simulink library "time_conversions_lib"  (R2016b)
settings: Solver=ode45  StartTime=0.0  StopTime=10.0  RelTol=1e-3  EnableMultiTasking=on
settings Model: Creator=Taylor  LastModifiedBy=Taylor
settings DataIOCC: LimitDataPoints=on
settings OptimizationCC: LifeSpan=inf
settings DebuggingCC: AllowSymbolicDim=off  SFUnexpectedBacktrackingDiag=warning  SFNoUnconditionalDefaultTransitionDiag=warning  SFExecutionAtInitializationDiag=none
settings GRTTargetCC: TargetLangStandard=C89/C90 (ANSI)  GeneratePreprocessorConditionals=Disable all
settings ConfigComp: CovMetricSettings=dw  CovHtmlReporting=on  CovSaveCumulativeToWorkspaceVar=on  CovSaveSingleToWorkspaceVar=on  CovExternalEMLEnable=off

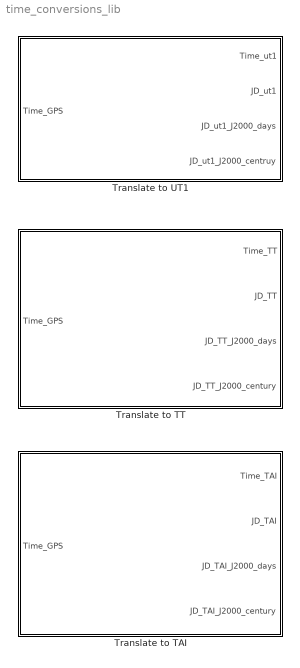
== system time_conversions_lib ==
  Translate to TAI : Subsystem
  Translate to TT : Subsystem
  Translate to UT1 : Subsystem

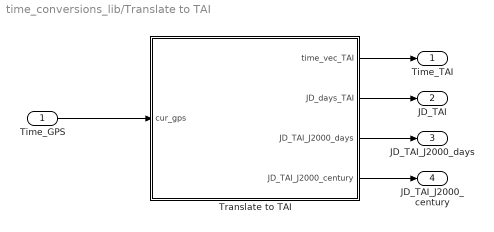
== system time_conversions_lib/Translate to TAI ==
  Time_GPS : Inport
  Translate to TAI : MATLAB Function  TreatAsAtomicUnit=on
  Time_TAI : Outport
  JD_TAI : Outport  Port=2
  JD_TAI_J2000_days : Outport  Port=3
  JD_TAI_J2000_century : Outport  Port=4
  wires:
  Translate to TAI/3(JD_TAI_J2000_days) -> JD_TAI_J2000_days/1
  Time_GPS/1 -> Translate to TAI/1(cur_gps)
  Translate to TAI/1(time_vec_TAI) -> Time_TAI/1
  Translate to TAI/2(JD_days_TAI) -> JD_TAI/1
  Translate to TAI/4(JD_TAI_J2000_century) -> JD_TAI_J2000_century/1

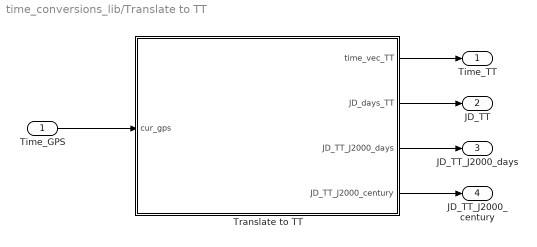
== system time_conversions_lib/Translate to TT ==
  Time_GPS : Inport
  Translate to TT : MATLAB Function  TreatAsAtomicUnit=on
  Time_TT : Outport
  JD_TT : Outport  Port=2
  JD_TT_J2000_days : Outport  Port=3
  JD_TT_J2000_century : Outport  Port=4
  wires:
  Time_GPS/1 -> Translate to TT/1(cur_gps)
  Translate to TT/1(time_vec_TT) -> Time_TT/1
  Translate to TT/2(JD_days_TT) -> JD_TT/1
  Translate to TT/3(JD_TT_J2000_days) -> JD_TT_J2000_days/1
  Translate to TT/4(JD_TT_J2000_century) -> JD_TT_J2000_century/1

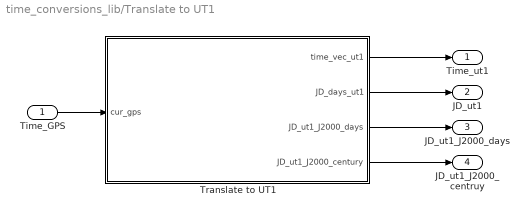
== system time_conversions_lib/Translate to UT1 ==
  Time_GPS : Inport
  Translate to UT1 : MATLAB Function  TreatAsAtomicUnit=on
  Time_ut1 : Outport
  JD_ut1 : Outport  Port=2
  JD_ut1_J2000_days : Outport  Port=3
  JD_ut1_J2000_centruy : Outport  Port=4
  wires:
  Translate to UT1/3(JD_ut1_J2000_days) -> JD_ut1_J2000_days/1
  Time_GPS/1 -> Translate to UT1/1(cur_gps)
  Translate to UT1/1(time_vec_ut1) -> Time_ut1/1
  Translate to UT1/4(JD_ut1_J2000_century) -> JD_ut1_J2000_centruy/1
  Translate to UT1/2(JD_days_ut1) -> JD_ut1/1

== matlab function time_conversions_lib/Translate to TAI/Translate to TAI ==
  data: cur_gps input; time_vec_TAI output; JD_days_TAI output; JD_TAI_J2000_days output; JD_TAI_J2000_century output
function [time_vec_TAI,JD_days_TAI,JD_TAI_J2000_days,JD_TAI_J2000_century] = fcn(cur_gps)
%#codegen

% ------ Prelim Stuff ------ %
% Account for leap seconds GPS --> TAI
gps2tai     = 19;

% sec --> JD conversion
sec2JD  = (0.0001/8.64); % JD/sec

feb = 28;
cal_days = [31, feb, 31, 30, 31, 30, 31, 31, 30, 31, 30, 31];

sec_in = cur_gps(1); week_in = cur_gps(2);
% -------------------------- %

% Translate GPS w-s to JD and Gregorian ymd-hms

JD_jan61980 = 2.444244500000000e+06;
JD_J2000    = 2451545;

JD_days_gps     = JD_jan61980 + 7*week_in + sec_in/3600/24;
JD_days_TAI     = JD_days_gps + sec2JD*gps2tai;

JD_TAI_J2000_days       = JD_days_TAI - JD_J2000;
JD_TAI_J2000_century    = (JD_days_TAI - 2451545)/36525;

T1900   = (JD_days_TAI - 2415019.5)/365.25;

year    = 1900 + floor(T1900);

leapyrs     = floor((year - 1900 - 1)*0.25);
days    = (JD_days_TAI - 2415019.5) - ((year - 1900)*365 + leapyrs );

if days < 1
    year = year - 1;
    leapyrs = floor((year - 1900 - 1)*0.25);
    days    = (JD_days_TAI - 2415019.5) - ((year - 1900)*365 + leapyrs );
end

if mod(year,4) == 0
    feb = 29;
end

dayofyear   = floor(days);

day     = 0;
i       = 0;

while day < dayofyear
    day = day + cal_days(i);
    i = i + 1;
end

month   = i - 1;

day_num = 0;
for i = 1:month
    day_num = day_num + cal_days(i);
end

day     = day - day_num;

tau     = 24*( day - dayofyear );

hour    = floor( tau );
min     = floor( 60*(tau - hour) );
sec     = 3600*( tau - hour - (min/60) );

% % Account for leap seconds GPS --> UT1
% sec = sec + gps2ut1;
% 
% if sec < 0
%     sec = mod(sec,60);
%     min = min - 1;
% end
% 
% if min < 0
%     min = mod(min,60);
%     hour = hour - 1;
% end
% 
% if hour < 0
%     hour = mod(hour,24);
%     day = day - 1;
% end
% 
% if day < 0
%     month = month - 1;
%     if month < 0
%         month = 12;
%         year = year - 1;
%     end
% end

time_vec_TAI = [year,month,day,hour,min,sec];

== matlab function time_conversions_lib/Translate to UT1/Translate to UT1 ==
  data: time_vec_ut1 output; cur_gps input; JD_days_ut1 output; JD_ut1_J2000_days output; JD_ut1_J2000_century output
function [time_vec_ut1,JD_days_ut1,JD_ut1_J2000_days,JD_ut1_J2000_century] = fcn(cur_gps)
%#codegen

% ------ Prelim Stuff ------ %
% Account for \Delta UT1 to get closest estimate to UT1
%   \Delta UT1 obtained from:
%       http://maia.usno.navy.mil/ser7/finals.daily
%   on Feb 24, 2017: 0.5236028

% Account for leap seconds GPS --> UT1
dut1 = 0.5236028;
gps2ut1     = dut1 - 18;

% sec --> JD conversion
sec2JD  = (0.0001/8.64); % JD/sec

feb = 28;
cal_days = [31, feb, 31, 30, 31, 30, 31, 31, 30, 31, 30, 31];

sec_in = cur_gps(1); week_in = cur_gps(2);
% --------------------------- %

% Translate GPS w-s to JD and Gregorian ymd-hms

JD_jan61980 = 2.444244500000000e+06;
JD_J2000    = 2451545;

JD_days_gps     = JD_jan61980 + 7*week_in + sec_in/3600/24;
JD_days_ut1     = JD_days_gps + sec2JD*gps2ut1;

JD_ut1_J2000_days       = JD_days_ut1 - JD_J2000;
JD_ut1_J2000_century    = (JD_days_ut1 - 2451545)/36525;

T1900   = (JD_days_ut1 - 2415019.5)/365.25;

year    = 1900 + floor(T1900);

leapyrs     = floor((year - 1900 - 1)*0.25);
days    = (JD_days_ut1 - 2415019.5) - ((year - 1900)*365 + leapyrs );

if days < 1
    year = year - 1;
    leapyrs = floor((year - 1900 - 1)*0.25);
    days    = (JD_days_ut1 - 2415019.5) - ((year - 1900)*365 + leapyrs );
end

if mod(year,4) == 0
    feb = 29;
end

dayofyear   = floor(days);

day     = 0;
i       = 0;

while day < dayofyear
    i   = i + 1;
    day = day + cal_days(i);
end

month   = i - 1;

day_num = 0;
for i = 1:month
    day_num = day_num + cal_days(i);
end

day     = day - day_num;

tau     = 24*( day - dayofyear );

hour    = floor( tau );
min     = floor( 60*(tau - hour) );
sec     = 3600*( tau - hour - (min/60) );

% % Account for leap seconds GPS --> UT1
% sec = sec + gps2ut1;
% 
% if sec < 0
%     sec = mod(sec,60);
%     min = min - 1;
% end
% 
% if min < 0
%     min = mod(min,60);
%     hour = hour - 1;
% end
% 
% if hour < 0
%     hour = mod(hour,24);
%     day = day - 1;
% end
% 
% if day < 0
%     month = month - 1;
%     if month < 0
%         month = 12;
%         year = year - 1;
%     end
% end

time_vec_ut1 = [year,month,day,hour,min,sec];

== matlab function time_conversions_lib/Translate to TT/Translate to TT ==
  data: cur_gps input; time_vec_TT output; JD_days_TT output; JD_TT_J2000_days output; JD_TT_J2000_century output
function [time_vec_TT,JD_days_TT,JD_TT_J2000_days,JD_TT_J2000_century] = fcn(cur_gps)
%#codegen

% ------ Prelim Stuff ------ %
% Account for \Delta UT1 to get closest estimate to UT1
%   \Delta UT1 obtained from:
%       http://maia.usno.navy.mil/ser7/finals.daily
%   on Feb 24, 2017: 0.5236028

% Account for leap seconds GPS --> TT
gps2tt     = 32.184 + (19);

% sec --> JD conversion
sec2JD  = (0.0001/8.64); % JD/sec

feb = 28;
cal_days = [31, feb, 31, 30, 31, 30, 31, 31, 30, 31, 30, 31];

sec_in = cur_gps(1); week_in = cur_gps(2);

% Translate GPS w-s to JD and Gregorian ymd-hms

JD_jan61980 = 2.444244500000000e+06;
JD_J2000    = 2451545;

JD_days_gps     = JD_jan61980 + 7*week_in + sec_in/3600/24;
JD_days_TT     = JD_days_gps + sec2JD*gps2tt;

JD_TT_J2000_days       = JD_days_TT - JD_J2000;
JD_TT_J2000_century    = (JD_days_TT - 2451545)/36525;

T1900   = (JD_days_TT - 2415019.5)/365.25;

year    = 1900 + floor(T1900);

leapyrs     = floor((year - 1900 - 1)*0.25);
days    = (JD_days_TT - 2415019.5) - ((year - 1900)*365 + leapyrs );

if days < 1
    year = year - 1;
    leapyrs = floor((year - 1900 - 1)*0.25);
    days    = (JD_days_TT - 2415019.5) - ((year - 1900)*365 + leapyrs );
end

if mod(year,4) == 0
    feb = 29;
end

dayofyear   = floor(days);

day     = 0;
i       = 0;

while day < dayofyear
    day = day + cal_days(i);
    i = i + 1;
end

month   = i - 1;

day_num = 0;
for i = 1:month
    day_num = day_num + cal_days(i);
end

day     = day - day_num;

tau     = 24*( day - dayofyear );

hour    = floor( tau );
min     = floor( 60*(tau - hour) );
sec     = 3600*( tau - hour - (min/60) );

% % Account for leap seconds GPS --> UT1
% sec = sec + gps2ut1;
% 
% if sec < 0
%     sec = mod(sec,60);
%     min = min - 1;
% end
% 
% if min < 0
%     min = mod(min,60);
%     hour = hour - 1;
% end
% 
% if hour < 0
%     hour = mod(hour,24);
%     day = day - 1;
% end
% 
% if day < 0
%     month = month - 1;
%     if month < 0
%         month = 12;
%         year = year - 1;
%     end
% end

time_vec_TT = [year,month,day,hour,min,sec];
